simulink model "mce"  (Simulink 6.5)
settings: Solver=ode45  StartTime=0.0  StopTime=10.0  RelTol=1e-3
libraries: cdsFilt x334, cdsMatrix x9, cdsSwitch x7, cdsWD x7, cdsMuxMatrix x5, dac x3, cdsEpicsOut x2, cdsParameters x1
(part 4 of 18)

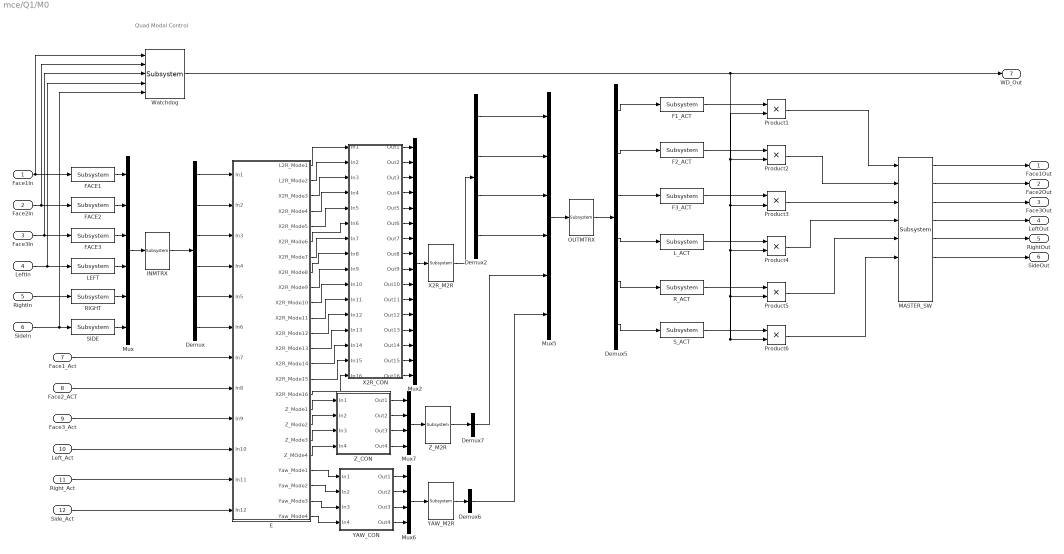
== system mce/Q1/M0 ==
  note: Quad Modal Control
  Face1In : Inport
  Face2In : Inport  Port=2
  Face3In : Inport  Port=3
  LeftIn : Inport  Port=4
  RightIn : Inport  Port=5
  SideIn : Inport  Port=6
  Face1_Act : Inport  Port=7
  Face2_ACT : Inport  Port=8
  Face3_Act : Inport  Port=9
  Left_Act : Inport  Port=10
  Right_Act : Inport  Port=11
  Side_Act : Inport  Port=12
  Demux : Demux  Outputs=6
  Demux2 : Demux
  Demux5 : Demux  Outputs=6
  Demux6 : Demux  Outputs=1
  Demux7 : Demux  Outputs=1
  E : Subsystem
  F1_ACT : cdsFilt/Subsystem  Tag=cdsFilt  Description=|  SystemSampleTime=-1
      | Purpose:                                                                                                                                                                                                                                  
      | Standard CDS IIR filter module.                                                                                                                                                                                                           
      |                                                                                                                                                                                                                                           
      | Operation:                                                                                                                                                                                                                                
      | Consists of 10 second order section IIR filters, plus a ramped gain stage. In FE code, also provides pre-defined test points and excitation channel inputs. The filter coefficients are defined in the LIGO system using the 'foton' tool.
      |                                                                                                                                                                                                                                           
      | Usage:                                                                                                                                                                                                                                    
      | Name the part with the desired filter module name.
      settings: AttributesFormatString=%<Tag>
  F2_ACT : cdsFilt/Subsystem  Tag=cdsFilt  Description=|  SystemSampleTime=-1
      | Purpose:                                                                                                                                                                                                                                  
      | Standard CDS IIR filter module.                                                                                                                                                                                                           
      |                                                                                                                                                                                                                                           
      | Operation:                                                                                                                                                                                                                                
      | Consists of 10 second order section IIR filters, plus a ramped gain stage. In FE code, also provides pre-defined test points and excitation channel inputs. The filter coefficients are defined in the LIGO system using the 'foton' tool.
      |                                                                                                                                                                                                                                           
      | Usage:                                                                                                                                                                                                                                    
      | Name the part with the desired filter module name.
      settings: AttributesFormatString=%<Tag>
  F3_ACT : cdsFilt/Subsystem  Tag=cdsFilt  Description=|  SystemSampleTime=-1
      | Purpose:                                                                                                                                                                                                                                  
      | Standard CDS IIR filter module.                                                                                                                                                                                                           
      |                                                                                                                                                                                                                                           
      | Operation:                                                                                                                                                                                                                                
      | Consists of 10 second order section IIR filters, plus a ramped gain stage. In FE code, also provides pre-defined test points and excitation channel inputs. The filter coefficients are defined in the LIGO system using the 'foton' tool.
      |                                                                                                                                                                                                                                           
      | Usage:                                                                                                                                                                                                                                    
      | Name the part with the desired filter module name.
      settings: AttributesFormatString=%<Tag>
  FACE1 : cdsFilt/Subsystem  Tag=cdsFilt  Description=|  SystemSampleTime=-1
      | Purpose:                                                                                                                                                                                                                                  
      | Standard CDS IIR filter module.                                                                                                                                                                                                           
      |                                                                                                                                                                                                                                           
      | Operation:                                                                                                                                                                                                                                
      | Consists of 10 second order section IIR filters, plus a ramped gain stage. In FE code, also provides pre-defined test points and excitation channel inputs. The filter coefficients are defined in the LIGO system using the 'foton' tool.
      |                                                                                                                                                                                                                                           
      | Usage:                                                                                                                                                                                                                                    
      | Name the part with the desired filter module name.
      settings: AttributesFormatString=%<Tag>
  FACE2 : cdsFilt/Subsystem  Tag=cdsFilt  Description=|  SystemSampleTime=-1
      | Purpose:                                                                                                                                                                                                                                  
      | Standard CDS IIR filter module.                                                                                                                                                                                                           
      |                                                                                                                                                                                                                                           
      | Operation:                                                                                                                                                                                                                                
      | Consists of 10 second order section IIR filters, plus a ramped gain stage. In FE code, also provides pre-defined test points and excitation channel inputs. The filter coefficients are defined in the LIGO system using the 'foton' tool.
      |                                                                                                                                                                                                                                           
      | Usage:                                                                                                                                                                                                                                    
      | Name the part with the desired filter module name.
      settings: AttributesFormatString=%<Tag>
  FACE3 : cdsFilt/Subsystem  Tag=cdsFilt  Description=|  SystemSampleTime=-1
      | Purpose:                                                                                                                                                                                                                                  
      | Standard CDS IIR filter module.                                                                                                                                                                                                           
      |                                                                                                                                                                                                                                           
      | Operation:                                                                                                                                                                                                                                
      | Consists of 10 second order section IIR filters, plus a ramped gain stage. In FE code, also provides pre-defined test points and excitation channel inputs. The filter coefficients are defined in the LIGO system using the 'foton' tool.
      |                                                                                                                                                                                                                                           
      | Usage:                                                                                                                                                                                                                                    
      | Name the part with the desired filter module name.
      settings: AttributesFormatString=%<Tag>
  INMTRX : cdsMuxMatrix/Subsystem  Tag=cdsMuxMatrix  Description=Any size matrix. Inputs and outputs must be connected using Mux and Demux parts.  SystemSampleTime=-1
      settings: AttributesFormatString=%<Tag>
  LEFT : cdsFilt/Subsystem  Tag=cdsFilt  Description=|  SystemSampleTime=-1
      | Purpose:                                                                                                                                                                                                                                  
      | Standard CDS IIR filter module.                                                                                                                                                                                                           
      |                                                                                                                                                                                                                                           
      | Operation:                                                                                                                                                                                                                                
      | Consists of 10 second order section IIR filters, plus a ramped gain stage. In FE code, also provides pre-defined test points and excitation channel inputs. The filter coefficients are defined in the LIGO system using the 'foton' tool.
      |                                                                                                                                                                                                                                           
      | Usage:                                                                                                                                                                                                                                    
      | Name the part with the desired filter module name.
      settings: AttributesFormatString=%<Tag>
  L_ACT : cdsFilt/Subsystem  Tag=cdsFilt  Description=|  SystemSampleTime=-1
      | Purpose:                                                                                                                                                                                                                                  
      | Standard CDS IIR filter module.                                                                                                                                                                                                           
      |                                                                                                                                                                                                                                           
      | Operation:                                                                                                                                                                                                                                
      | Consists of 10 second order section IIR filters, plus a ramped gain stage. In FE code, also provides pre-defined test points and excitation channel inputs. The filter coefficients are defined in the LIGO system using the 'foton' tool.
      |                                                                                                                                                                                                                                           
      | Usage:                                                                                                                                                                                                                                    
      | Name the part with the desired filter module name.
      settings: AttributesFormatString=%<Tag>
  MASTER_SW : cdsSwitch/Subsystem  SystemSampleTime=-1
  Mux : Mux  Inputs=6
  Mux2 : Mux  Inputs=16
  Mux5 : Mux  Inputs=6
  Mux6 : Mux
  Mux7 : Mux
  OUTMTRX : cdsMuxMatrix/Subsystem  Tag=cdsMuxMatrix  Description=Any size matrix. Inputs and outputs must be connected using Mux and Demux parts.  SystemSampleTime=-1
      settings: AttributesFormatString=%<Tag>
  Product{1..6} (6 alike) : Product  RndMeth=Zero
  RIGHT : cdsFilt/Subsystem  Tag=cdsFilt  Description=|  SystemSampleTime=-1
      | Purpose:                                                                                                                                                                                                                                  
      | Standard CDS IIR filter module.                                                                                                                                                                                                           
      |                                                                                                                                                                                                                                           
      | Operation:                                                                                                                                                                                                                                
      | Consists of 10 second order section IIR filters, plus a ramped gain stage. In FE code, also provides pre-defined test points and excitation channel inputs. The filter coefficients are defined in the LIGO system using the 'foton' tool.
      |                                                                                                                                                                                                                                           
      | Usage:                                                                                                                                                                                                                                    
      | Name the part with the desired filter module name.
      settings: AttributesFormatString=%<Tag>
  R_ACT : cdsFilt/Subsystem  Tag=cdsFilt  Description=|  SystemSampleTime=-1
      | Purpose:                                                                                                                                                                                                                                  
      | Standard CDS IIR filter module.                                                                                                                                                                                                           
      |                                                                                                                                                                                                                                           
      | Operation:                                                                                                                                                                                                                                
      | Consists of 10 second order section IIR filters, plus a ramped gain stage. In FE code, also provides pre-defined test points and excitation channel inputs. The filter coefficients are defined in the LIGO system using the 'foton' tool.
      |                                                                                                                                                                                                                                           
      | Usage:                                                                                                                                                                                                                                    
      | Name the part with the desired filter module name.
      settings: AttributesFormatString=%<Tag>
  SIDE : cdsFilt/Subsystem  Tag=cdsFilt  Description=|  SystemSampleTime=-1
      | Purpose:                                                                                                                                                                                                                                  
      | Standard CDS IIR filter module.                                                                                                                                                                                                           
      |                                                                                                                                                                                                                                           
      | Operation:                                                                                                                                                                                                                                
      | Consists of 10 second order section IIR filters, plus a ramped gain stage. In FE code, also provides pre-defined test points and excitation channel inputs. The filter coefficients are defined in the LIGO system using the 'foton' tool.
      |                                                                                                                                                                                                                                           
      | Usage:                                                                                                                                                                                                                                    
      | Name the part with the desired filter module name.
      settings: AttributesFormatString=%<Tag>
  S_ACT : cdsFilt/Subsystem  Tag=cdsFilt  Description=|  SystemSampleTime=-1
      | Purpose:                                                                                                                                                                                                                                  
      | Standard CDS IIR filter module.                                                                                                                                                                                                           
      |                                                                                                                                                                                                                                           
      | Operation:                                                                                                                                                                                                                                
      | Consists of 10 second order section IIR filters, plus a ramped gain stage. In FE code, also provides pre-defined test points and excitation channel inputs. The filter coefficients are defined in the LIGO system using the 'foton' tool.
      |                                                                                                                                                                                                                                           
      | Usage:                                                                                                                                                                                                                                    
      | Name the part with the desired filter module name.
      settings: AttributesFormatString=%<Tag>
  Watchdog : cdsWD/Subsystem  Description=cdsWD  SystemSampleTime=-1
      settings: AttributesFormatString=%<Description>
  X2R_CON : Subsystem
  X2R_M2R : cdsMuxMatrix/Subsystem  Tag=cdsMuxMatrix  Description=Any size matrix. Inputs and outputs must be connected using Mux and Demux parts.  SystemSampleTime=-1
      settings: AttributesFormatString=%<Tag>
  YAW_CON : Subsystem
  YAW_M2R : cdsMuxMatrix/Subsystem  Tag=cdsMuxMatrix  Description=Any size matrix. Inputs and outputs must be connected using Mux and Demux parts.  SystemSampleTime=-1
      settings: AttributesFormatString=%<Tag>
  Z_CON : Subsystem
  Z_M2R : cdsMuxMatrix/Subsystem  Tag=cdsMuxMatrix  Description=Any size matrix. Inputs and outputs must be connected using Mux and Demux parts.  SystemSampleTime=-1
      settings: AttributesFormatString=%<Tag>
  Face1Out : Outport
  Face2Out : Outport  Port=2
  Face3Out : Outport  Port=3
  LeftOut : Outport  Port=4
  RightOut : Outport  Port=5
  SideOut : Outport  Port=6
  WD_Out : Outport  Port=7
  wires:
  E/1(L2R_Mode1) -> X2R_CON/1(In1)
  E/2(L2R_Mode2) -> X2R_CON/2(In2)
  E/3(X2R_Mode3) -> X2R_CON/3(In3)
  E/4(X2R_Mode4) -> X2R_CON/4(In4)
  E/5(X2R_Mode5) -> X2R_CON/5(In5)
  E/6(X2R_Mode6) -> X2R_CON/6(In6)
  E/7(X2R_Mode7) -> X2R_CON/7(In7)
  E/8(X2R_Mode8) -> X2R_CON/8(In8)
  E/9(X2R_Mode9) -> X2R_CON/9(In9)
  E/10(X2R_Mode10) -> X2R_CON/10(In10)
  E/11(X2R_Mode11) -> X2R_CON/11(In11)
  E/12(X2R_Mode12) -> X2R_CON/12(In12)
  E/13(X2R_Mode13) -> X2R_CON/13(In13)
  E/14(X2R_Mode14) -> X2R_CON/14(In14)
  E/15(X2R_Mode15) -> X2R_CON/15(In15)
  E/16(X2R_Mode16) -> X2R_CON/16(In16)
  E/17(Z_Mode1) -> Z_CON/1(In1)
  E/18(Z_Mode2) -> Z_CON/2(In2)
  E/19(Z_Mode3) -> Z_CON/3(In3)
  E/20(Z_MOde4) -> Z_CON/4(In4)
  E/21(Yaw_Mode1) -> YAW_CON/1(In1)
  E/22(Yaw_Mode2) -> YAW_CON/2(In2)
  E/23(Yaw_Mode3) -> YAW_CON/3(In3)
  E/24(Yaw_Mode4) -> YAW_CON/4(In4)
  Mux/1 -> INMTRX/1
  INMTRX/1 -> Demux/1
  Demux/1 -> E/1(In1)
  Demux/2 -> E/2(In2)
  Demux/3 -> E/3(In3)
  Demux/4 -> E/4(In4)
  Demux/5 -> E/5(In5)
  Demux/6 -> E/6(In6)
  FACE1/1 -> Mux/1
  FACE2/1 -> Mux/2
  FACE3/1 -> Mux/3
  LEFT/1 -> Mux/4
  RIGHT/1 -> Mux/5
  SIDE/1 -> Mux/6
  Mux2/1 -> X2R_M2R/1
  X2R_M2R/1 -> Demux2/1
  Mux6/1 -> YAW_M2R/1
  YAW_M2R/1 -> Demux6/1
  Mux7/1 -> Z_M2R/1
  Z_M2R/1 -> Demux7/1
  X2R_CON/1(Out1) -> Mux2/1
  X2R_CON/2(Out2) -> Mux2/2
  X2R_CON/3(Out3) -> Mux2/3
  X2R_CON/4(Out4) -> Mux2/4
  X2R_CON/5(Out5) -> Mux2/5
  X2R_CON/6(Out6) -> Mux2/6
  X2R_CON/7(Out7) -> Mux2/7
  X2R_CON/8(Out8) -> Mux2/8
  X2R_CON/9(Out9) -> Mux2/9
  X2R_CON/10(Out10) -> Mux2/10
  X2R_CON/11(Out11) -> Mux2/11
  X2R_CON/12(Out12) -> Mux2/12
  X2R_CON/13(Out13) -> Mux2/13
  X2R_CON/14(Out14) -> Mux2/14
  X2R_CON/15(Out15) -> Mux2/15
  X2R_CON/16(Out16) -> Mux2/16
  Z_CON/1(Out1) -> Mux7/1
  Z_CON/2(Out2) -> Mux7/2
  Z_CON/3(Out3) -> Mux7/3
  Z_CON/4(Out4) -> Mux7/4
  Demux7/1 -> Mux5/5
  YAW_CON/1(Out1) -> Mux6/1
  YAW_CON/2(Out2) -> Mux6/2
  YAW_CON/3(Out3) -> Mux6/3
  YAW_CON/4(Out4) -> Mux6/4
  Demux6/1 -> Mux5/6
  Face3In/1 -> FACE3/1, Watchdog/3
  LeftIn/1 -> LEFT/1, Watchdog/4
  RightIn/1 -> RIGHT/1
  SideIn/1 -> SIDE/1, Watchdog/5
  Watchdog/1 -> Product6/2, Product5/2, Product4/2, Product3/2, Product2/2, Product1/2, WD_Out/1
  F1_ACT/1 -> Product1/1
  F2_ACT/1 -> Product2/1
  F3_ACT/1 -> Product3/1
  L_ACT/1 -> Product4/1
  R_ACT/1 -> Product5/1
  S_ACT/1 -> Product6/1
  Product1/1 -> MASTER_SW/1
  Product2/1 -> MASTER_SW/2
  Product3/1 -> MASTER_SW/3
  Product4/1 -> MASTER_SW/4
  Product5/1 -> MASTER_SW/5
  Product6/1 -> MASTER_SW/6
  Face1In/1 -> Watchdog/1, FACE1/1
  Face2In/1 -> Watchdog/2, FACE2/1
  MASTER_SW/1 -> Face1Out/1
  MASTER_SW/2 -> Face2Out/1
  MASTER_SW/3 -> Face3Out/1
  MASTER_SW/4 -> LeftOut/1
  MASTER_SW/5 -> RightOut/1
  MASTER_SW/6 -> SideOut/1
  Mux5/1 -> OUTMTRX/1
  OUTMTRX/1 -> Demux5/1
  Demux2/1 -> Mux5/1
  Demux2/2 -> Mux5/2
  Demux2/3 -> Mux5/3
  Demux5/1 -> F1_ACT/1
  Demux5/2 -> F2_ACT/1
  Demux5/3 -> F3_ACT/1
  Demux5/4 -> L_ACT/1
  Demux5/5 -> R_ACT/1
  Demux5/6 -> S_ACT/1
  Demux2/4 -> Mux5/4
  Face1_Act/1 -> E/7(In7)
  Face2_ACT/1 -> E/8(In8)
  Face3_Act/1 -> E/9(In9)
  Left_Act/1 -> E/10(In10)
  Right_Act/1 -> E/11(In11)
  Side_Act/1 -> E/12(In12)
